simulink model "control"  (R2023b)
settings: Solver=VariableStepAuto  StartTime=0.0  StopTime=10.0  RelTol=1e-3
libraries: fuzblock x1, simulink x1
settings Model: Creator=Lenovo  LastModifiedBy=Lenovo

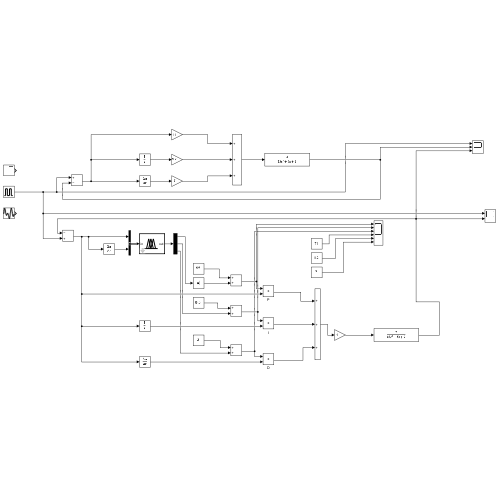
[thumbnail: Simulink's stored preview of the top-level diagram]
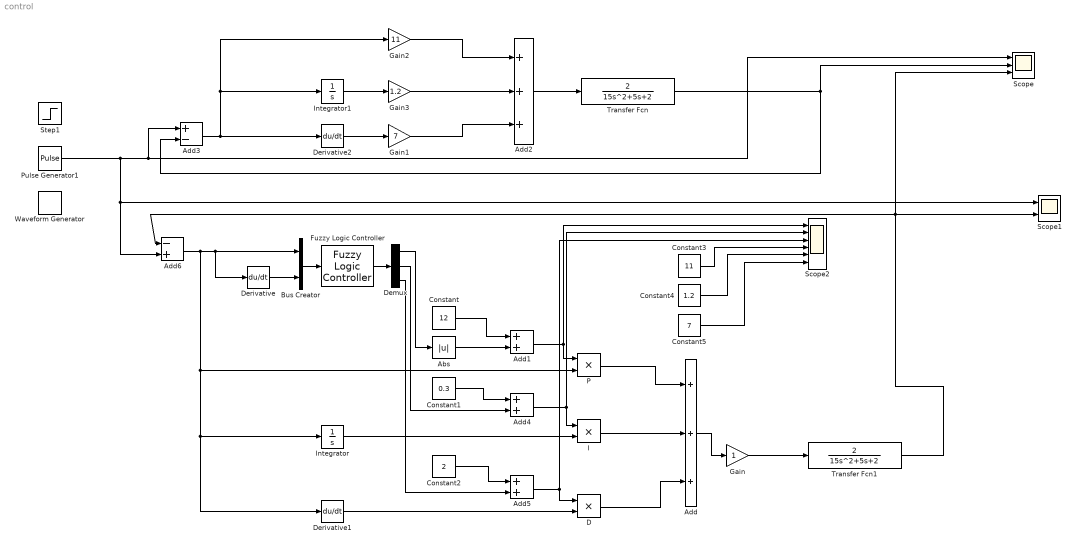
== system control ==
  Abs : Abs  ZeroCross=off  SaturateOnIntegerOverflow=off
  Add : Sum  Inputs=+++
  Add1 : Sum
  Add2 : Sum  Inputs=+++
  Add3 : Sum  Inputs=+-
  Add4 : Sum
  Add5 : Sum
  Add6 : Sum  Inputs=-+
  Bus Creator : BusCreator  Inputs=2
  Constant : Constant  Value=12
  Constant1 : Constant  Value=0.3
  Constant2 : Constant  Value=2
  Constant3 : Constant  Value=11
  Constant4 : Constant  Value=1.2
  Constant5 : Constant  Value=7
  D : Product
  Demux : Demux  Outputs=3
  Derivative : Derivative
  Derivative1 : Derivative
  Derivative2 : Derivative
  Fuzzy Logic Controller : fuzblock/Fuzzy Logic  Controller  FIS='fuzzy.fis'  OutputSampleNumber=101  DataType=double  FuzzifiedInputs=off  RuleFiringStrengths=off  RuleOutputs=off  AggregatedOutputs=off  SimulateUsing=Interpreted execution  OutOfRangeInputValueMessage=warning  NoRuleFiredMessage=warning  EmptyOutputFuzzySetMessage=warning
  Gain : Gain
  Gain1 : Gain  Gain=7
  Gain2 : Gain  Gain=11
  Gain3 : Gain  Gain=1.2
  I : Product
  Integrator : Integrator
  Integrator1 : Integrator  UpperSaturationLimit=10  LowerSaturationLimit=-10
  P : Product
  Pulse Generator1 : DiscretePulseGenerator  PulseType=Time based  Amplitude=21  Period=10  PulseWidth=50
  Scope : Scope  NumInputPorts=3
  Scope1 : Scope  NumInputPorts=2
  Scope2 : Scope  NumInputPorts=6
  Step1 : Step  After=3  SampleTime=0
  Transfer Fcn : TransferFcn  Numerator=[2]  Denominator=[15 5 2]
  Transfer Fcn1 : TransferFcn  Numerator=[2]  Denominator=[15 5 2]
  Waveform Generator : simulink/Sources/Waveform Generator  OutMin=[]  OutMax=[]  OutDataTypeStr=double  SelectedSignal=1  BlockNames=MultiportSwitch_e3df3653d217406  SampleTime=0.1
  wires:
  Add3/1 -> Gain2/1, Integrator1/1, Derivative2/1
  Derivative2/1 -> Gain1/1
  Bus Creator/1 -> Fuzzy Logic Controller/1
  Add6/1 -> Derivative1/1, Integrator/1, P/2, Derivative/1, Bus Creator/1
  Derivative/1 -> Bus Creator/2
  Fuzzy Logic Controller/1 -> Demux/1
  Demux/1 -> Abs/1
  Demux/3 -> Add5/2
  Derivative1/1 -> D/2
  Integrator/1 -> I/2
  P/1 -> Add/1
  Add/1 -> Gain/1
  Gain/1 -> Transfer Fcn1/1
  Abs/1 -> Add1/2
  Add1/1 -> P/1, Scope2/1
  Constant/1 -> Add1/1
  Transfer Fcn1/1 -> Scope/3, Add6/1, Scope1/2
  D/1 -> Add/3
  Integrator1/1 -> Gain3/1
  Gain2/1 -> Add2/1
  Add2/1 -> Transfer Fcn/1
  Pulse Generator1/1 -> Add6/2, Scope1/1, Add3/1, Scope/1
  Transfer Fcn/1 -> Add3/2, Scope/2
  Demux/2 -> Add4/2
  Add5/1 -> Scope2/3, D/1
  Constant2/1 -> Add5/1
  I/1 -> Add/2
  Constant1/1 -> Add4/1
  Add4/1 -> Scope2/2, I/1
  Gain1/1 -> Add2/3
  Gain3/1 -> Add2/2
  Constant3/1 -> Scope2/4
  Constant4/1 -> Scope2/5
  Constant5/1 -> Scope2/6
